simulink model "untitled"  (R2022b)
settings: Solver=VariableStepAuto  StartTime=0.0  StopTime=10.0  RelTol=1e-3
settings Model: Creator=richa  LastModifiedBy=richa

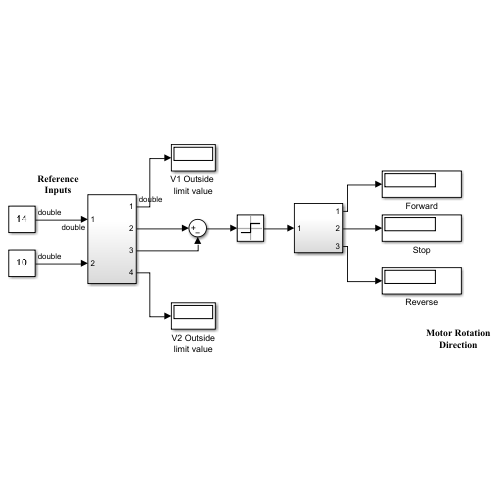
[thumbnail: Simulink's stored preview of the top-level diagram]
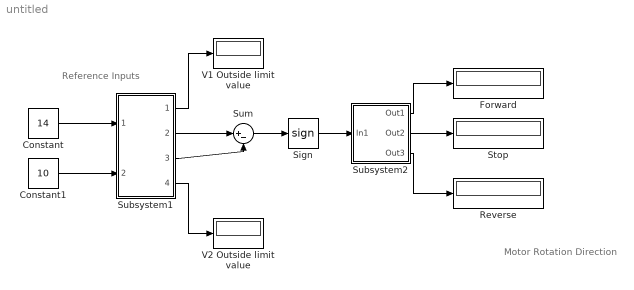
== system untitled ==
  note: Reference
      | Inputs
  note: Motor Rotation
      | Direction
  Constant : Constant  Value=14
  Constant1 : Constant  Value=10
  Forward : Display
  Reverse : Display
  Sign : Signum
  Stop : Display
  Subsystem1 : Subsystem
  Subsystem2 : Subsystem
  Sum : Sum  Inputs=|+-  InputSameDT=on  SaturateOnIntegerOverflow=on  OutDataTypeStr=Inherit: Same as first input
  V1 Outside limit value : Display
  V2 Outside limit value : Display
  wires:
  Sign/1 -> Subsystem2/1(In1)
  Subsystem2/2(Out2) -> Stop/1
  Subsystem1/1(Out1) -> V1 Outside limit value/1
  Constant/1 -> Subsystem1/1(Input)
  Constant1/1 -> Subsystem1/2(Input1)
  Sum/1 -> Sign/1
  Subsystem1/3(Out3) -> Sum/2
  Subsystem1/4(Out4) -> V2 Outside limit value/1
  Subsystem1/2(Out2) -> Sum/1
  Subsystem2/1(Out1) -> Forward/1
  Subsystem2/3(Out3) -> Reverse/1

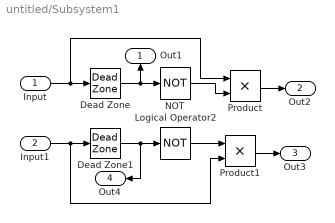
== system untitled/Subsystem1 ==
  Input : Inport
  Input1 : Inport  Port=2
  Dead Zone : DeadZone  LowerValue=5  UpperValue=15
  Dead Zone1 : DeadZone  LowerValue=5  UpperValue=15
  Logical Operator2 : Logic  Operator=NOT
  NOT : Logic  Operator=NOT  IconShape=distinctive  AllPortsSameDT=off  OutDataTypeStr=boolean
  Product : Product  InputSameDT=on  RndMeth=Zero  SaturateOnIntegerOverflow=on  OutDataTypeStr=Inherit: Same as first input
  Product1 : Product  InputSameDT=on  RndMeth=Zero  SaturateOnIntegerOverflow=on  OutDataTypeStr=Inherit: Same as first input
  Out1 : Outport
  Out2 : Outport  Port=2
  Out3 : Outport  Port=3
  Out4 : Outport  Port=4
  wires:
  NOT/1 -> Product/2
  Logical Operator2/1 -> Product1/1
  Input/1 -> Dead Zone/1, Product/1
  Input1/1 -> Dead Zone1/1, Product1/2
  Dead Zone/1 -> NOT/1, Out1/1
  Dead Zone1/1 -> Logical Operator2/1, Out4/1
  Product/1 -> Out2/1
  Product1/1 -> Out3/1

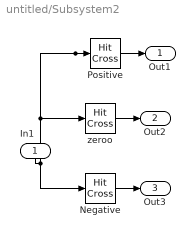
== system untitled/Subsystem2 ==
  In1 : Inport
  Negative : HitCross  HitCrossingOffset=-1
  Positive : HitCross  HitCrossingOffset=1
  zeroo : HitCross
  Out1 : Outport
  Out2 : Outport  Port=2
  Out3 : Outport  Port=3
  wires:
  In1/1 -> Negative/1, Positive/1, zeroo/1
  Positive/1 -> Out1/1
  zeroo/1 -> Out2/1
  Negative/1 -> Out3/1
